simulink model "main"  (R2018a)
settings: Solver=VariableStepAuto  StartTime=0.0  StopTime=100  FixedStep=0.01  RelTol=1e-3  EnableMultiTasking=on
InitFcn:
  | %run constants
StopFcn:
  | %run runafter
values from neighbouring files (symbols this model uses):
  dt = 0.01    [constants.m]    (also in state_estimatation.m)
  dt_noise = 0.1    [constants.m]
  eul_0 = [tendeg tendeg tendeg]    [constants.m]
  inertia = [2500 0 0 ... (first row only)    [constants.m]
  n = tracking * n_magnitude    [constants.m]
  phi_D = -2434    [constants.m]
  phi_I = -21    [constants.m]
  phi_P = -465    [constants.m]
  pm_0 = [0 0 0]    [constants.m]
  pqr_noise = [p_noise q_noise r_noise]    [constants.m]
  Psi_D = -30035    [constants.m]
  Psi_I = -460    [constants.m]
  Psi_P = -7886    [constants.m]
  T_d = Td_on * [0.001 0.001 0.001]    [constants.m]
  theta_D = -2213    [constants.m]
  theta_I = -28.5    [constants.m]
  theta_P = -568    [constants.m]
  use_xhat = false    [constants.m]
libraries: simulink x3, shared6dofsys x2, sharedTrackingLibrary x1
settings Model: PacingRate=1000  Creator=Matt  LastModifiedBy=matth
settings SolverCC: AutoInsertRateTranBlk=on
settings DataIOCC: SaveOutput=off  SaveTime=off
settings OptimizationCC: DefaultParameterBehavior=Inlined  InlineInvariantSignals=on  EnhancedBackFolding=on  PassReuseOutputArgsAs=Individual arguments  StateBitsets=on  DataBitsets=on  ZeroExternalMemoryAtStartup=off  ZeroInternalMemoryAtStartup=off  NoFixptDivByZeroProtection=on  LifeSpan=1  OptimizeBlockOrder=speed  DifferentSizesBufferReuse=on
settings DebuggingCC: ParameterTunabilityLossMsg=error
settings HardwareCC: ProdBitPerPointer=32  ProdBitPerSizeT=32  ProdBitPerPtrDiffT=32  ProdLargestAtomicFloat=None  ProdIntDivRoundTo=Floor  ProdWordSize=32  ProdHWDeviceType=Generic->Custom
settings SFSimCC: MATLABDynamicMemAlloc=off
settings RTWCC: SystemTargetFile=ert.tlc  TLCOptions=-p0  GenCodeOnly=on  TemplateMakefile=ert_default_tmf  GenerateReport=on  RTWVerbose=off  IncludeHyperlinkInReport=on  LaunchReport=on  GenerateTraceInfo=on  GenerateTraceReport=on  GenerateTraceReportSl=on  GenerateTraceReportSf=on  GenerateTraceReportEml=on
settings CodeAppCC: ForceParamTrailComments=on  IgnoreCustomStorageClasses=off  OperatorAnnotations=on  SimulinkDataObjDesc=on  SFDataObjDesc=on  CustomSymbolStrGlobalVar=rt$N$M  CustomSymbolStrType=$N$M  CustomSymbolStrFcn=$N$M$F  CustomSymbolStrMacro=$N$M  InsertBlockDesc=on
settings ERTTargetCC: TargetLangStandard=C99 (ISO)  CodeReplacementLibrary=ISO_C  GenerateSampleERTMain=on  IncludeMdlTerminateFcn=off  SuppressErrorStatus=on  SupportAbsoluteTime=off  SupportNonFinite=off  SupportComplex=off  PurelyIntegerCode=on  InlinedParameterPlacement=NonHierarchical  RootIOFormat=Structure reference  ERTCustomFileTemplate=example_file_process.tlc

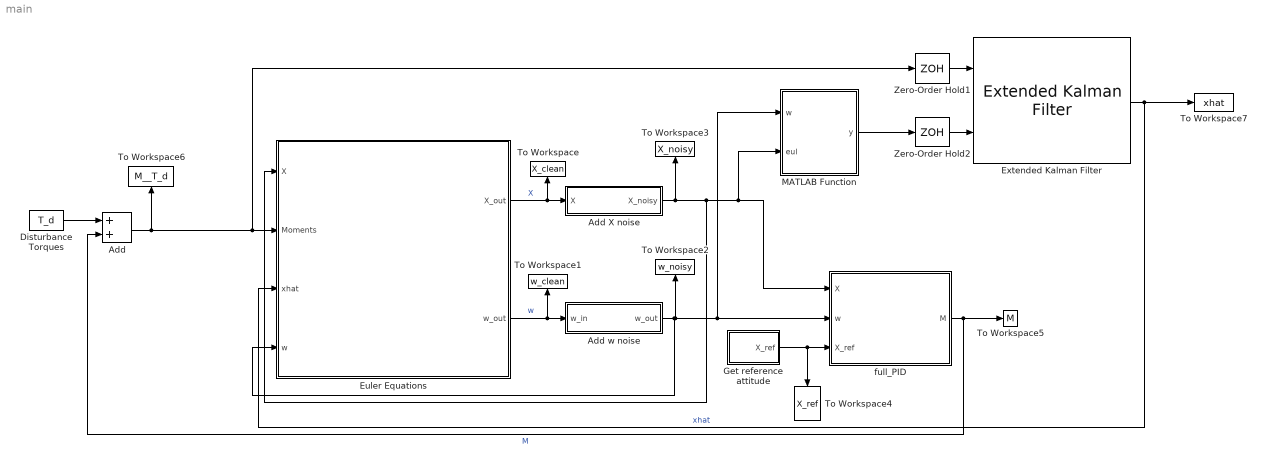
== system main ==
  Add : Sum
  "Add X noise " : Subsystem
  Add w noise : Subsystem
  Disturbance Torques : Constant  Value=T_d
  Euler Equations : Subsystem
  Extended Kalman Filter : sharedTrackingLibrary/Extended Kalman Filter  StateTransitionFcn=state_estimatation  HasStateTransitionJacobianFcn=off  HasAdditiveProcessNoise=Additive  ProcessNoise=state_covar  HasTimeVaryingProcessNoise=off  HasStateTransitionFcnExtraArgument=1  InitialState=state_init  InitialStateCovariance=init_covar  MeasurementFcn1=measure_func  HasMeasurementJacobianFcn1=off  HasMeasurementEnablePort1=off  HasAdditiveMeasurementNoise1=Additive  MeasurementNoise1=measure_covar  HasTimeVaryingMeasurementNoise1=off  HasMeasurementFcnExtraArgument1=0  MeasurementFcn2=myMeasurementFcn  HasMeasurementJacobianFcn2=off  HasMeasurementEnablePort2=off  HasAdditiveMeasurementNoise2=Additive  MeasurementNoise2=1  HasTimeVaryingMeasurementNoise2=off  HasMeasurementFcnExtraArgument2=0  MeasurementFcn3=myMeasurementFcn  HasMeasurementJacobianFcn3=off  HasMeasurementEnablePort3=off  HasAdditiveMeasurementNoise3=Additive  MeasurementNoise3=1  HasTimeVaryingMeasurementNoise3=off  HasMeasurementFcnExtraArgument3=0  MeasurementFcn4=myMeasurementFcn  HasMeasurementJacobianFcn4=off  HasMeasurementEnablePort4=off  HasAdditiveMeasurementNoise4=Additive  MeasurementNoise4=1  HasTimeVaryingMeasurementNoise4=off  HasMeasurementFcnExtraArgument4=0  MeasurementFcn5=myMeasurementFcn  HasMeasurementJacobianFcn5=off  HasMeasurementEnablePort5=off  HasAdditiveMeasurementNoise5=Additive  MeasurementNoise5=1  HasTimeVaryingMeasurementNoise5=off  HasMeasurementFcnExtraArgument5=0  EnableMultirate=off  StateTransitionFcnSampleTime=1  MeasurementFcn1SampleTime=1  MeasurementFcn2SampleTime=1  MeasurementFcn3SampleTime=1  MeasurementFcn4SampleTime=1  MeasurementFcn5SampleTime=1  UseCurrentEstimator=off  OutputStateCovariance=off  DataType=double  SampleTime=dt  NumberOfMeasurements=1
      settings: SourceProductName=Control System Toolbox  SourceProductBaseCode=CT
  Get reference attitude : Subsystem
  MATLAB Function : MATLAB Function  TreatAsAtomicUnit=on
  To Workspace : ToWorkspace  VariableName=X_clean  SaveFormat=Timeseries  SampleTime=-1
      settings: AttributesFormatString=Save X_clean
  To Workspace1 : ToWorkspace  VariableName=w_clean  SaveFormat=Timeseries  SampleTime=-1
      settings: AttributesFormatString=Save w_clean
  To Workspace2 : ToWorkspace  VariableName=w_noisy  SaveFormat=Timeseries  SampleTime=-1
      settings: AttributesFormatString=Save w_noisy
  To Workspace3 : ToWorkspace  VariableName=X_noisy  SaveFormat=Timeseries  SampleTime=-1
      settings: AttributesFormatString=Save X_noisy
  To Workspace4 : ToWorkspace  VariableName=X_ref  SaveFormat=Timeseries  SampleTime=-1
      settings: AttributesFormatString=Save X_ref
  To Workspace5 : ToWorkspace  VariableName=M  SaveFormat=Timeseries  SampleTime=-1
      settings: AttributesFormatString=Save M
  To Workspace6 : ToWorkspace  VariableName=M__T_d  SaveFormat=Timeseries  SampleTime=-1
      settings: AttributesFormatString=Save M__T_d
  To Workspace7 : ToWorkspace  VariableName=xhat  SampleTime=-1
      settings: AttributesFormatString=Save xhat  Save2DSignal=2-D array (concatenate along first dimension)
  Zero-Order Hold1 : ZeroOrderHold  SampleTime=dt
      settings: AttributesFormatString=Zero-order hold
  Zero-Order Hold2 : ZeroOrderHold  SampleTime=dt
      settings: AttributesFormatString=Zero-order hold
  "full_PID " : Subsystem
  wires:
  Euler Equations/1(X_out) -> "Add X noise "/1(X), To Workspace/1  "X"
  "full_PID "/1(M) -> Add/2, To Workspace5/1  "M"
  Disturbance Torques/1 -> Add/1
  Add/1 -> Zero-Order Hold1/1, Euler Equations/2(Moments), To Workspace6/1
  Euler Equations/2(w_out) -> Add w noise/1(w_in), To Workspace1/1  "w"
  MATLAB Function/1(y) -> Zero-Order Hold2/1
  Zero-Order Hold1/1 -> Extended Kalman Filter/1
  Zero-Order Hold2/1 -> Extended Kalman Filter/2
  Get reference attitude/1(X_ref) -> "full_PID "/3(X_ref), To Workspace4/1
  Add w noise/1(w_out) -> MATLAB Function/1(w), "full_PID "/2(w), To Workspace2/1, Euler Equations/4("w ")
  "Add X noise "/1(X_noisy) -> "full_PID "/1(X), MATLAB Function/2(eul), Euler Equations/1(X), To Workspace3/1
  Extended Kalman Filter/1 -> Euler Equations/3(xhat), To Workspace7/1  "xhat"

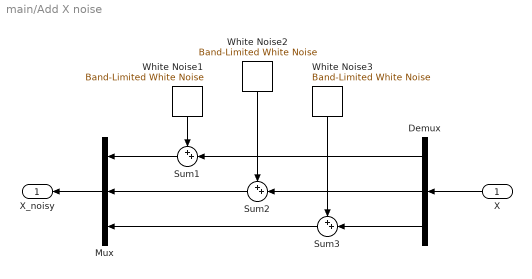
== system main/Add X noise  ==
  X : Inport
  Demux : Demux  Outputs=3
  Mux : Mux  Inputs=3
  Sum1 : Sum  Inputs=++|
  Sum2 : Sum  Inputs=++|
  Sum3 : Sum  Inputs=++|
  White Noise1 : simulink/Sources/Band-Limited White Noise  Cov=noise_att_mag  Ts=dt_noise  seed=[23340]
  White Noise2 : simulink/Sources/Band-Limited White Noise  Cov=noise_att_mag  Ts=dt_noise  seed=[23341]
  White Noise3 : simulink/Sources/Band-Limited White Noise  Cov=noise_att_mag  Ts=dt_noise  seed=[23342]
  X_noisy : Outport
  wires:
  Demux/2 -> Sum2/2
  Demux/3 -> Sum3/2
  Sum2/1 -> Mux/2
  Sum3/1 -> Mux/3
  Sum1/1 -> Mux/1
  White Noise3/1 -> Sum3/1
  Demux/1 -> Sum1/2
  Mux/1 -> X_noisy/1
  X/1 -> Demux/1
  White Noise2/1 -> Sum2/1
  White Noise1/1 -> Sum1/1

== system main/Add w noise ==
  w_in : Inport
  Add : Sum
  w_bias : Constant  Value=pqr_noise
  w_out : Outport
  wires:
  w_in/1 -> Add/2
  w_bias/1 -> Add/1
  Add/1 -> w_out/1

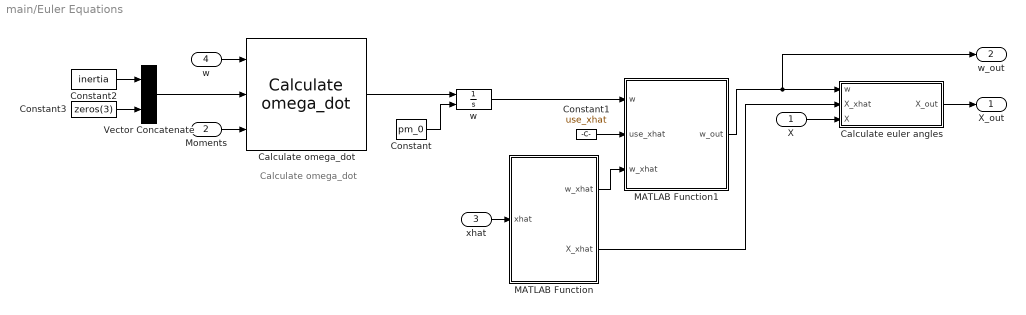
== system main/Euler Equations ==
  note: Calculate omega_dot
  X : Inport
  Moments : Inport  Port=2  Unit=N*m  PortDimensions=3
  xhat : Inport  Port=3
  "w " : Inport  Port=4
  Calculate euler angles : Subsystem
  Calculate omega_dot : shared6dofsys/Calculate omega_dot  aMode=aMode
      settings: SourceProductName=Aerospace Blockset  SourceProductBaseCode=AE
  Constant : Constant  Value=pm_0
  Constant1 : Constant  Value=use_xhat
  Constant2 : Constant  Value=inertia  OutDataTypeStr=Inherit: Inherit via back propagation
  Constant3 : Constant  Value=zeros(3)
  MATLAB Function : MATLAB Function  TreatAsAtomicUnit=on
  MATLAB Function1 : MATLAB Function  TreatAsAtomicUnit=on
  Vector Concatenate : Concatenate  Mode=Multidimensional array
  w : Integrator  InitialConditionSource=external  InitialCondition=pm_0
  X_out : Outport  Unit=rad
  w_out : Outport  Port=2
  wires:
  Calculate euler angles/1(X_out) -> X_out/1
  Moments/1 -> Calculate omega_dot/3
  Vector Concatenate/1 -> Calculate omega_dot/2
  Constant/1 -> w/2
  MATLAB Function1/1(w_out) -> w_out/1, Calculate euler angles/1(w)
  xhat/1 -> MATLAB Function/1(xhat)
  MATLAB Function/1(w_xhat) -> MATLAB Function1/3(w_xhat)
  w/1 -> MATLAB Function1/1(w)
  Constant1/1 -> MATLAB Function1/2(use_xhat)
  MATLAB Function/2(X_xhat) -> Calculate euler angles/2(X_xhat)
  Calculate omega_dot/1 -> w/1
  X/1 -> Calculate euler angles/3("X ")
  "w "/1 -> Calculate omega_dot/1
  Constant3/1 -> Vector Concatenate/2
  Constant2/1 -> Vector Concatenate/1

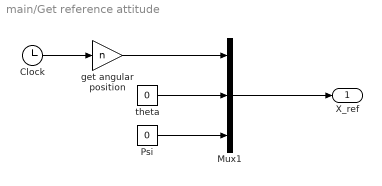
== system main/Get reference attitude ==
  Clock : Clock
  Mux1 : Mux  Inputs=3
  "Psi " : Constant  Value=0
  get angular position : Gain  Gain=n
  theta : Constant  Value=0
  X_ref : Outport
  wires:
  Mux1/1 -> X_ref/1
  "Psi "/1 -> Mux1/3
  theta/1 -> Mux1/2
  get angular position/1 -> Mux1/1
  Clock/1 -> get angular position/1

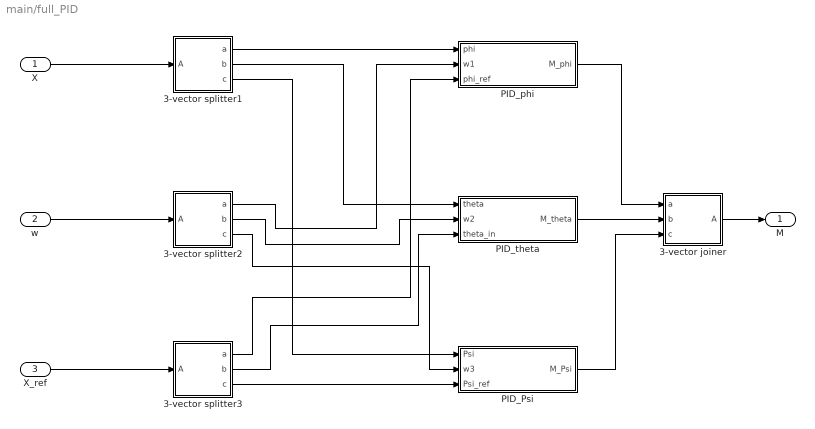
== system main/full_PID  ==
  X : Inport
  w : Inport  Port=2
  X_ref : Inport  Port=3
  3-vector joiner : Subsystem
  3-vector splitter1 : Subsystem
  "3-vector splitter2 " : Subsystem
  3-vector splitter3 : Subsystem
  PID_Psi : Subsystem
  PID_phi : Subsystem
  PID_theta : Subsystem
  M : Outport  InitialOutput=0
  wires:
  X/1 -> 3-vector splitter1/1(A)
  w/1 -> "3-vector splitter2 "/1(A)
  X_ref/1 -> 3-vector splitter3/1(A)
  3-vector splitter1/1(a) -> PID_phi/1(phi)
  3-vector splitter1/2(b) -> PID_theta/1(theta)
  3-vector splitter1/3(c) -> PID_Psi/1(Psi)
  "3-vector splitter2 "/1(a) -> PID_phi/2(w1)
  "3-vector splitter2 "/2(b) -> PID_theta/2(w2)
  "3-vector splitter2 "/3(c) -> PID_Psi/2(w3)
  3-vector splitter3/1(a) -> PID_phi/3(phi_ref)
  3-vector splitter3/2(b) -> PID_theta/3(theta_in)
  3-vector splitter3/3(c) -> PID_Psi/3("Psi_ref ")
  PID_theta/1("M_theta ") -> 3-vector joiner/2(b)
  PID_phi/1(M_phi) -> 3-vector joiner/1(a)
  PID_Psi/1(M_Psi) -> 3-vector joiner/3(c)
  3-vector joiner/1(A) -> M/1

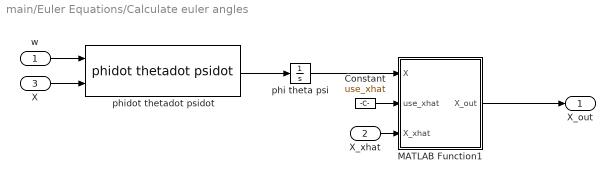
== system main/Euler Equations/Calculate euler angles ==
  w : Inport
  X_xhat : Inport  Port=2
  "X " : Inport  Port=3
  Constant : Constant  Value=use_xhat
  MATLAB Function1 : MATLAB Function  TreatAsAtomicUnit=on
  phi theta psi : Integrator  InitialCondition=eul_0  WrapState=on
  phidot thetadot psidot : shared6dofsys/DCM & Euler Angles (Euler)/phidot thetadot psidot
      settings: SourceProductName=Aerospace Blockset  SourceProductBaseCode=AE
  X_out : Outport
  wires:
  w/1 -> phidot thetadot psidot/1
  phidot thetadot psidot/1 -> phi theta psi/1
  MATLAB Function1/1(X_out) -> X_out/1
  phi theta psi/1 -> MATLAB Function1/1(X)
  X_xhat/1 -> MATLAB Function1/3(X_xhat)
  Constant/1 -> MATLAB Function1/2(use_xhat)
  "X "/1 -> phidot thetadot psidot/2

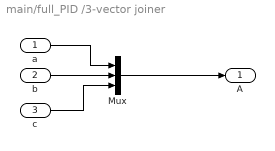
== system main/full_PID /3-vector joiner ==
  a : Inport
  b : Inport  Port=2
  c : Inport  Port=3
  Mux : Mux  Inputs=3
  A : Outport
  wires:
  c/1 -> Mux/3
  a/1 -> Mux/1
  b/1 -> Mux/2
  Mux/1 -> A/1

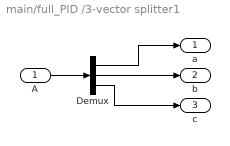
== system main/full_PID /3-vector splitter1 ==
  A : Inport
  Demux : Demux  Outputs=3
  a : Outport
  b : Outport  Port=2
  c : Outport  Port=3
  wires:
  Demux/3 -> c/1
  Demux/2 -> b/1
  Demux/1 -> a/1
  A/1 -> Demux/1

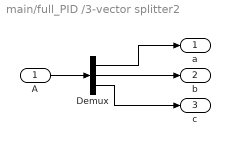
== system main/full_PID /3-vector splitter2  ==
  A : Inport
  Demux : Demux  Outputs=3
  a : Outport
  b : Outport  Port=2
  c : Outport  Port=3
  wires:
  Demux/3 -> c/1
  Demux/2 -> b/1
  Demux/1 -> a/1
  A/1 -> Demux/1

== system main/full_PID /3-vector splitter3 ==
  A : Inport
  Demux : Demux  Outputs=3
  a : Outport
  b : Outport  Port=2
  c : Outport  Port=3
  wires:
  Demux/3 -> c/1
  Demux/2 -> b/1
  Demux/1 -> a/1
  A/1 -> Demux/1

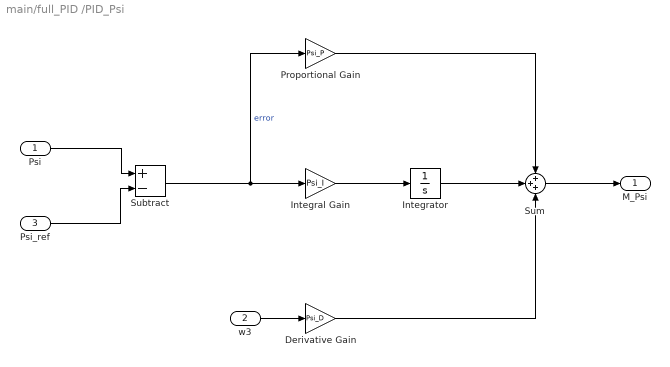
== system main/full_PID /PID_Psi ==
  Psi : Inport
  w3 : Inport  Port=2
  "Psi_ref " : Inport  Port=3
  Derivative Gain : Gain  Gain=Psi_D
  Integral Gain : Gain  Gain=Psi_I
  Integrator : Integrator
  Proportional Gain : Gain  Gain=Psi_P
  Subtract : Sum  Inputs=+-
  Sum : Sum  Inputs=+++
  M_Psi : Outport
  wires:
  Psi/1 -> Subtract/1
  "Psi_ref "/1 -> Subtract/2
  Subtract/1 -> Integral Gain/1, Proportional Gain/1  "error"
  Integral Gain/1 -> Integrator/1
  Proportional Gain/1 -> Sum/1
  Integrator/1 -> Sum/2
  w3/1 -> Derivative Gain/1
  Derivative Gain/1 -> Sum/3
  Sum/1 -> M_Psi/1

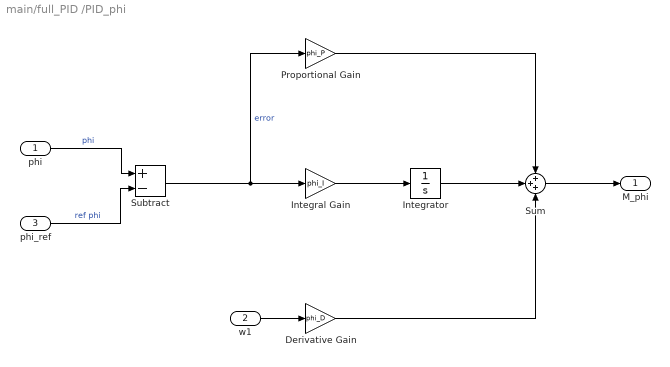
== system main/full_PID /PID_phi ==
  phi : Inport
  w1 : Inport  Port=2
  phi_ref : Inport  Port=3
  Derivative Gain : Gain  Gain=phi_D
  Integral Gain : Gain  Gain=phi_I
  Integrator : Integrator
  Proportional Gain : Gain  Gain=phi_P
  Subtract : Sum  Inputs=+-
  Sum : Sum  Inputs=+++
  M_phi : Outport
  wires:
  phi/1 -> Subtract/1  "phi"
  phi_ref/1 -> Subtract/2  "ref phi"
  Subtract/1 -> Integral Gain/1, Proportional Gain/1  "error"
  Integral Gain/1 -> Integrator/1
  Proportional Gain/1 -> Sum/1
  Integrator/1 -> Sum/2
  w1/1 -> Derivative Gain/1
  Derivative Gain/1 -> Sum/3
  Sum/1 -> M_phi/1

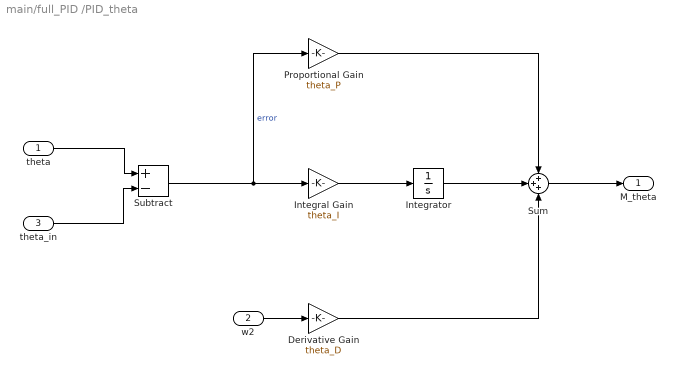
== system main/full_PID /PID_theta ==
  theta : Inport
  w2 : Inport  Port=2
  theta_in : Inport  Port=3
  Derivative Gain : Gain  Gain=theta_D
  Integral Gain : Gain  Gain=theta_I
  Integrator : Integrator
  Proportional Gain : Gain  Gain=theta_P
  Subtract : Sum  Inputs=+-
  Sum : Sum  Inputs=+++
  "M_theta " : Outport
  wires:
  theta/1 -> Subtract/1
  theta_in/1 -> Subtract/2
  Subtract/1 -> Integral Gain/1, Proportional Gain/1  "error"
  Integral Gain/1 -> Integrator/1
  Proportional Gain/1 -> Sum/1
  Integrator/1 -> Sum/2
  w2/1 -> Derivative Gain/1
  Derivative Gain/1 -> Sum/3
  Sum/1 -> "M_theta "/1

== matlab function main/Euler Equations/MATLAB Function ==
  data: w_xhat output; X_xhat output; xhat input
function [w_xhat, X_xhat]= xhat2X_w(xhat)

X_xhat = [xhat(1); xhat(2); xhat(3)];
w_xhat = [xhat(4); xhat(5); xhat(6)];

end

== matlab function main/MATLAB Function ==
  data: w input; eul input; y output
function y = get_state(w, eul)

y = [eul(1) eul(2) eul(3) w(1) w(2) w(3)];
end

== matlab function main/Euler Equations/MATLAB Function1 ==
  data: w input; use_xhat input; w_xhat input; w_out output
function w_out = check_w_xhat(w, use_xhat, w_xhat)

use_xhat = false;
if use_xhat == true
    w_out = w_xhat;
else
    w_out = w;
end

end

== matlab function main/Euler Equations/Calculate euler angles/MATLAB Function1 ==
  data: X input; use_xhat input; X_xhat input; X_out output
function X_out = check_X_xhat(X, use_xhat, X_xhat)

if use_xhat == true
    X_out = X_xhat;
else
    X_out = X;
end

end
